simulink model "EST"  (R2025a)
settings: Solver=FixedStepAuto  StartTime=0.0  StopTime=31536000  FixedStep=deltat  MaxStep=0.05  RelTol=1e-3
values from neighbouring files (symbols this model uses):
  A_tank = 6*pi*r_tank^2    [preprocessing.m]
  C_s = m_ads*c_ads + m_w_min*c_w + m_tank*c_tank    [preprocessing.m]
  deltaH = 2.579E6*unit("J")/unit("kg")    [preprocessing.m]
  efficiencyBattery = 0.90    (= 0.9)    [preprocessing.m]
  efficiencyHeater = 1.00    (= 1)    [preprocessing.m]
  EStorageInitial = 2.0*unit("kWh")    [preprocessing.m]
  k_0 = (15*D_0)/(d_p/2)^2    [preprocessing.m]
  m_eq = m_w_max    [preprocessing.m]
  m_w_0 = m_w_min    [preprocessing.m]
  m_w_min = X_min*m_ads    [preprocessing.m]
  Max_Capacity_J = volumes_m3(k) * energy_density * conversion_factor    [optimalization.m]    (also in preprocessing.m = EStorageMax)
  R = 8.314*unit("J")/(unit("mol")*unit("K"))    [preprocessing.m]
  R_cable = L_cable*Rprime_cable    [preprocessing.m]
  T_ambient = (8+273.15)*unit("K")    [preprocessing.m]
  T_s_0 = T_ambient    [preprocessing.m]
  T_w = (50+273.15)*unit("K")    [preprocessing.m]
  U_tank = 1 / (1/h_inside + t_wall/k_steel + 1/h_outside)    [preprocessing.m]
  UA_pipe = U_pipe*A_pipe    [preprocessing.m]
  V_system = 400    [preprocessing.m]
settings Model: Creator=joche  LastModifiedBy=20253351
settings DataIOCC: SaveFormat=Array  SaveOutput=off  ReturnWorkspaceOutputs=off
settings OptimizationCC: ReuseModelBlockBuffer=off
settings ModelReferenceCC: EnableRefExpFcnMdlSchedulingChecks=on
settings RTWCC: GPUComputeCapability=3.5

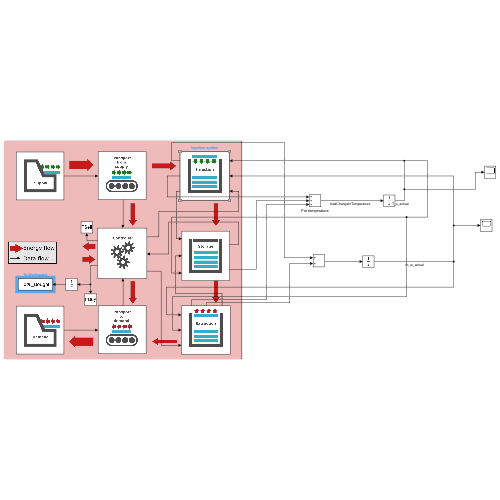
[thumbnail: Simulink's stored preview of the top-level diagram]
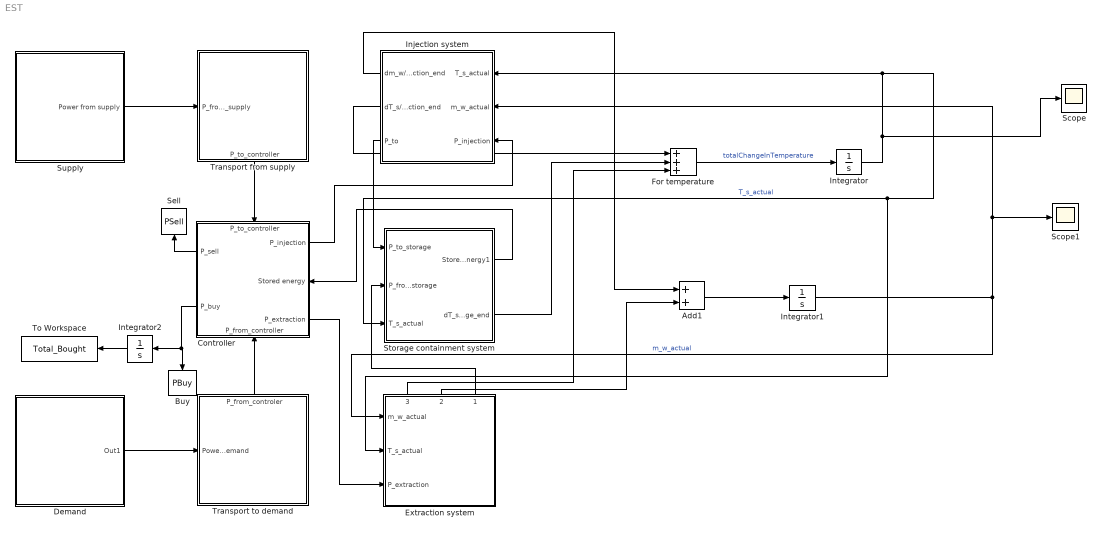
== system EST ==
  Add1 : Sum
  Buy : ToWorkspace  VariableName=PBuy  SampleTime=-1
  Controller : Subsystem
      settings: PortSchema="{\"entries\":[{\"content\":{\"sides\":[{\"content\":{\"connectorIds\":[\"Out3\",\"Out4\"]},\"type\":\"ConnectorPlacement.EquallySpacedRectSide\",\"uuid\":\"4daf33ce-c96a-4783-b5c4-228eed953e01\"},{\"content\":{\"connectorIds\":[\"Out1\",\"In3\",\"Out2\"],\"side\":\"RIGHT\"},\"type\":\"ConnectorPlacement.EquallySpacedRectSide\",\"uuid\":\"e9942e50-8467-4af8-b79b-80636cbc76e5\"},{\"content\":{\"connectorIds\":[\"In1\"],\"side\":\"TOP\"},\"type\":\"ConnectorPlacement.EquallySpacedRectSide\",\"uuid\":\"f315e931-d69b-4751-b712-f89c6c81baeb\"},{\"content\":{\"connectorIds\":[\"In2\"],\"side\":\"BOTTOM\"},\"type\":\"ConnectorPlacement.EquallySpacedRectSide\",\"uuid\":\"44715ee6-5cd5-4669-bcb9-5ed7c869bdb3\"}]},\"type\":\"ConnectorPlacement.EquallySpacedConnector\",\"uuid\":\"fff48899-944b-4064-b7d7-ecc12144fb48\"}],\"packageUris\":[\"http://schema.mathworks.com/mf0/Connector/R2020b\"],\"version\":\"1.0\"}"
      mask Display: image('$imagefile'); % Use "Edit Image" on toolstrip to change.
  Demand : Subsystem
      mask Display: image('$imagefile'); % Use "Edit Image" on toolstrip to change.
  Extraction system : Subsystem
      settings: PortSchema="{\"entries\":[{\"content\":{\"sides\":[{\"content\":{},\"type\":\"ConnectorPlacement.EquallySpacedRectSide\",\"uuid\":\"05c5933d-55fc-4e06-853f-fc26d42905f9\"},{\"content\":{\"connectorIds\":[\"In1\",\"In2\",\"In3\"],\"side\":\"RIGHT\"},\"type\":\"ConnectorPlacement.EquallySpacedRectSide\",\"uuid\":\"327426c5-31d5-498b-a2bd-83e49353408c\"},{\"content\":{\"side\":\"TOP\"},\"type\":\"ConnectorPlacement.EquallySpacedRectSide\",\"uuid\":\"55306cf3-a3de-4385-a5ae-b8600ecdd5a2\"},{\"content\":{\"connectorIds\":[\"Out1\",\"Out2\",\"Out3\"],\"side\":\"BOTTOM\"},\"type\":\"ConnectorPlacement.EquallySpacedRectSide\",\"uuid\":\"08fcc9c3-40d3-4ac6-b914-dfeef6039ffb\"}]},\"type\":\"ConnectorPlacement.EquallySpacedConnector\",\"uuid\":\"cb35d5ba-e8c6-462c-b7b2-fe8356d4b0a1\"}],\"packageUris\":[\"http://schema.mathworks.com/mf0/Connector/R2020b\"],\"version\":\"1.0\"}"
      mask Display: image('$imagefile'); % Use "Edit Image" on toolstrip to change.
  For temperature : Sum  Inputs=+++
  Injection system : Subsystem
      mask Display: image('$imagefile'); % Use "Edit Image" on toolstrip to change.
  Integrator : Integrator  InitialCondition=T_s_0
  Integrator1 : Integrator  InitialCondition=m_w_0
  Integrator2 : Integrator
  Scope : Scope
      settings: ActiveDisplayYMinimum=-1  ActiveDisplayYMaximum=1  DataLoggingVariableName=ScopeData7
  Scope1 : Scope
      settings: ActiveDisplayYMinimum=-895.99568542877842  ActiveDisplayYMaximum=10043.823661162089  DataLoggingVariableName=ScopeData8
  Sell : ToWorkspace  VariableName=PSell  SampleTime=-1
  Storage containment system : Subsystem
      mask Display: image('$imagefile'); % Use "Edit Image" on toolstrip to change.
  Supply : Subsystem
      mask Display: image('$imagefile'); % Use "Edit Image" on toolstrip to change.
  To Workspace : ToWorkspace  VariableName=Total_Bought  SaveFormat=Timeseries  SampleTime=-1
  Transport from supply : Subsystem
      settings: PortSchema="{\"entries\":[{\"content\":{\"sides\":[{\"content\":{\"connectorIds\":[\"In1\"]},\"type\":\"ConnectorPlacement.EquallySpacedRectSide\",\"uuid\":\"31329006-3d36-4d93-9c44-7503a515d397\"},{\"content\":{\"connectorIds\":[],\"side\":\"RIGHT\"},\"type\":\"ConnectorPlacement.EquallySpacedRectSide\",\"uuid\":\"aba139c7-f9b6-4881-a56b-a4cbbedacd88\"},{\"content\":{\"connectorIds\":[],\"side\":\"TOP\"},\"type\":\"ConnectorPlacement.EquallySpacedRectSide\",\"uuid\":\"e683eb73-7a35-4160-9c39-da83856a6278\"},{\"content\":{\"connectorIds\":[\"Out1\"],\"side\":\"BOTTOM\"},\"type\":\"ConnectorPlacement.EquallySpacedRectSide\",\"uuid\":\"1170dd18-447c-437f-9043-6812c2877331\"}]},\"type\":\"ConnectorPlacement.EquallySpacedConnector\",\"uuid\":\"804af608-1d70-444f-af69-e05f19bf98f3\"}],\"packageUris\":[\"http://schema.mathworks.com/mf0/Connector/R2020b\"],\"version\":\"1.0\"}"
      mask Display: image('$imagefile'); % Use "Edit Image" on toolstrip to change.
  Transport to demand : Subsystem
      settings: PortSchema="{\"entries\":[{\"content\":{\"sides\":[{\"content\":{\"connectorIds\":[\"In1\"]},\"type\":\"ConnectorPlacement.EquallySpacedRectSide\",\"uuid\":\"31329006-3d36-4d93-9c44-7503a515d397\"},{\"content\":{\"connectorIds\":[],\"side\":\"RIGHT\"},\"type\":\"ConnectorPlacement.EquallySpacedRectSide\",\"uuid\":\"aba139c7-f9b6-4881-a56b-a4cbbedacd88\"},{\"content\":{\"connectorIds\":[\"Out1\"],\"side\":\"TOP\"},\"type\":\"ConnectorPlacement.EquallySpacedRectSide\",\"uuid\":\"e683eb73-7a35-4160-9c39-da83856a6278\"},{\"content\":{\"connectorIds\":[],\"side\":\"BOTTOM\"},\"type\":\"ConnectorPlacement.EquallySpacedRectSide\",\"uuid\":\"c378138f-7233-4483-870c-40a69b3495ee\"}]},\"type\":\"ConnectorPlacement.EquallySpacedConnector\",\"uuid\":\"804af608-1d70-444f-af69-e05f19bf98f3\"}],\"packageUris\":[\"http://schema.mathworks.com/mf0/Connector/R2020b\"],\"version\":\"1.0\"}"
      mask Display: image('$imagefile'); % Use "Edit Image" on toolstrip to change.
  wires:
  Supply/1(Power from supply) -> Transport from supply/1(P_from_supply)
  Transport from supply/1(P_to_controller) -> Controller/1(P_to_controller)
  Transport to demand/1(P_from_controler) -> Controller/2(P_from_controller)
  Demand/1(Out1) -> Transport to demand/1(Power to demand)
  Controller/3(P_sell) -> Sell/1
  Controller/2(P_extraction) -> Extraction system/1(P_extraction)
  Injection system/1(P_to) -> Storage containment system/1(P_to_storage)
  Extraction system/1(P_from_storage) -> Storage containment system/2(P_from_storage)
  Storage containment system/1(Stored energy1) -> Controller/3(Stored energy)
  Controller/1(P_injection) -> Injection system/1(P_injection)
  Controller/4(P_buy) -> Integrator2/1, Buy/1
  Injection system/2(dT_s/dt_injection_end) -> For temperature/1
  Storage containment system/2(dT_s/dt_storage_end) -> For temperature/2
  Extraction system/3(dT_s/dt_end_extraction) -> For temperature/3
  For temperature/1 -> Integrator/1  "totalChangeInTemperature"
  Integrator/1 -> Scope/1, Injection system/3(T_s_actual), Extraction system/2(T_s_actual), Storage containment system/3(T_s_actual)  "T_s_actual"
  Injection system/3(dm_w/dt_injection_end) -> Add1/1
  Extraction system/2(dm_w/dt_end_extraction) -> Add1/2
  Add1/1 -> Integrator1/1
  Integrator1/1 -> Scope1/1, Injection system/2(m_w_actual), Extraction system/3(m_w_actual)  "m_w_actual"
  Integrator2/1 -> To Workspace/1

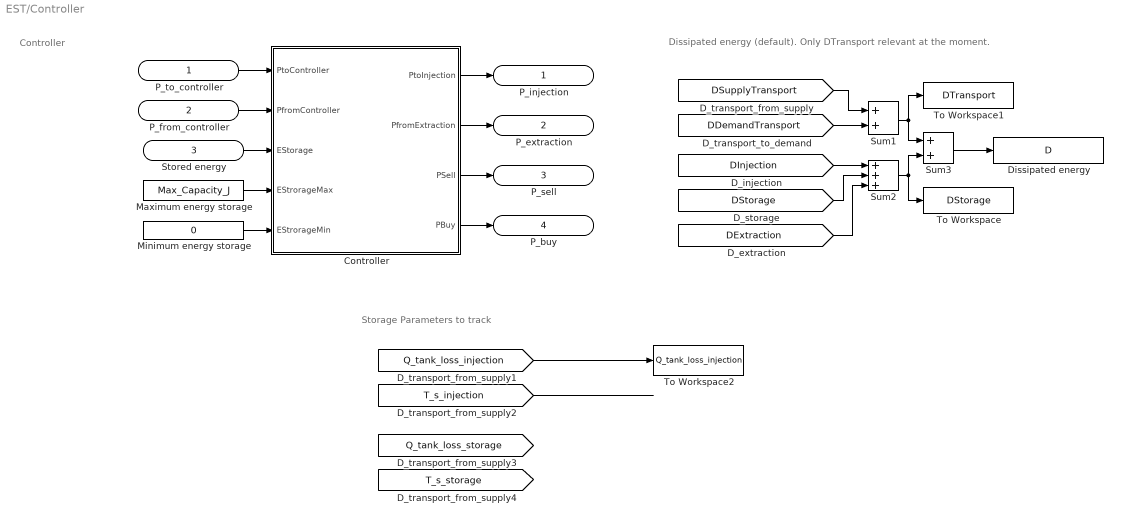
== system EST/Controller ==
  note: Dissipated energy (default). Only DTransport relevant at the moment.
  note: Controller
  note: Storage Parameters to track
  P_to_controller : Inport
  P_from_controller : Inport  Port=2
  Stored energy : Inport  Port=3
  Controller : MATLAB Function  TreatAsAtomicUnit=on
  Dissipated energy : ToWorkspace  VariableName=D  SampleTime=-1
  Maximum energy storage : Constant  Value=Max_Capacity_J
  Minimum energy storage : Constant  Value=0
  Sum1 : Sum
  Sum2 : Sum  Inputs=+++
  Sum3 : Sum
  To Workspace : ToWorkspace  VariableName=DStorage  SampleTime=-1
  To Workspace1 : ToWorkspace  VariableName=DTransport  SampleTime=-1
  To Workspace2 : ToWorkspace  VariableName=Q_tank_loss_injection  SaveFormat=Timeseries  SampleTime=-1
  P_injection : Outport
  P_extraction : Outport  Port=2
  P_sell : Outport  Port=3
  P_buy : Outport  Port=4
  wires:
  P_from_controller/1 -> Controller/2(PfromController)
  Controller/2(PfromExtraction) -> P_extraction/1
  Controller/3(PSell) -> P_sell/1
  Controller/4(PBuy) -> P_buy/1
  Minimum energy storage/1 -> Controller/5(EStrorageMin)
  Maximum energy storage/1 -> Controller/4(EStrorageMax)
  P_to_controller/1 -> Controller/1(PtoController)
  Controller/1(PtoInjection) -> P_injection/1
  Stored energy/1 -> Controller/3(EStorage)
  [DDemandTransport] -> Sum1/2
  [DSupplyTransport] -> Sum1/1
  [DInjection] -> Sum2/1
  [DStorage] -> Sum2/2
  [DExtraction] -> Sum2/3
  Sum2/1 -> To Workspace/1, Sum3/2
  Sum1/1 -> To Workspace1/1, Sum3/1
  Sum3/1 -> Dissipated energy/1
  [Q_tank_loss_injection] -> To Workspace2/1
  [T_s_injection] -> ?

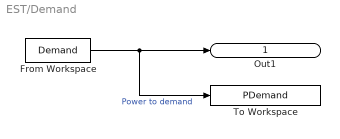
== system EST/Demand ==
  From Workspace : FromWorkspace  VariableName=Demand  OutputAfterFinalValue=Setting to zero
  To Workspace : ToWorkspace  VariableName=PDemand  SampleTime=-1
  Out1 : Outport
  wires:
  From Workspace/1 -> To Workspace/1, Out1/1  "Power to demand"

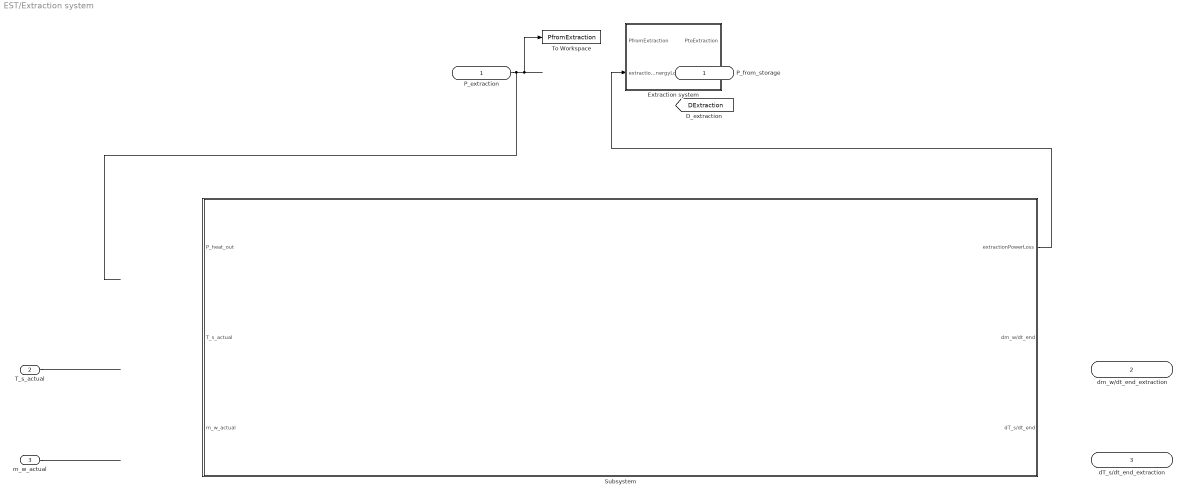
== system EST/Extraction system ==
  P_extraction : Inport
  T_s_actual : Inport  Port=2
  m_w_actual : Inport  Port=3
  Extraction system : MATLAB Function  TreatAsAtomicUnit=on
  Subsystem : Subsystem
  To Workspace : ToWorkspace  VariableName=PfromExtraction  SampleTime=-1
  P_from_storage : Outport
  dm_w/dt_end_extraction : Outport  Port=2
  dT_s/dt_end_extraction : Outport  Port=3
  tag scope: DExtraction=global
  wires:
  P_extraction/1 -> To Workspace/1
  ? -> P_from_storage/1
  ? -> [DExtraction]
  Subsystem/1(extractionPowerLoss) -> Extraction system/2(extractionEnergyLoss)
  ? -> dm_w/dt_end_extraction/1
  ? -> dT_s/dt_end_extraction/1
  T_s_actual/1 -> ?
  m_w_actual/1 -> ?

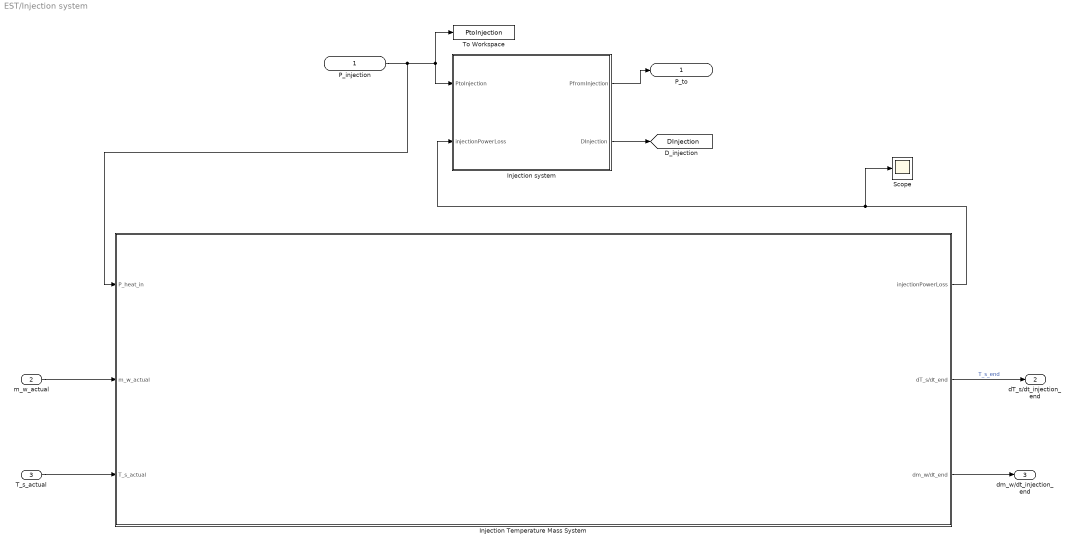
== system EST/Injection system ==
  P_injection : Inport
  m_w_actual : Inport  Port=2
  T_s_actual : Inport  Port=3
  Injection Temperature Mass System : Subsystem
  Injection system : MATLAB Function  TreatAsAtomicUnit=on
  Scope : Scope
      settings: ActiveDisplayYMinimum=-7184.0347360498881  ActiveDisplayYMaximum=5973.1294987784431  DataLoggingVariableName=ScopeData9
  To Workspace : ToWorkspace  VariableName=PtoInjection  SampleTime=-1
  P_to : Outport
  dT_s/dt_injection_end : Outport  Port=2
  dm_w/dt_injection_end : Outport  Port=3
  tag scope: DInjection=global
  wires:
  P_injection/1 -> Injection Temperature Mass System/1(P_heat_in), Injection system/1(PtoInjection), To Workspace/1
  Injection system/2(DInjection) -> [DInjection]
  Injection system/1(PfromInjection) -> P_to/1
  Injection Temperature Mass System/1(injectionPowerLoss) -> Scope/1, Injection system/2(injectionPowerLoss)
  Injection Temperature Mass System/3(dm_w/dt_end) -> dm_w/dt_injection_end/1
  Injection Temperature Mass System/2(dT_s/dt_end) -> dT_s/dt_injection_end/1  "T_s_end"
  m_w_actual/1 -> Injection Temperature Mass System/2(m_w_actual)
  T_s_actual/1 -> Injection Temperature Mass System/3(T_s_actual)

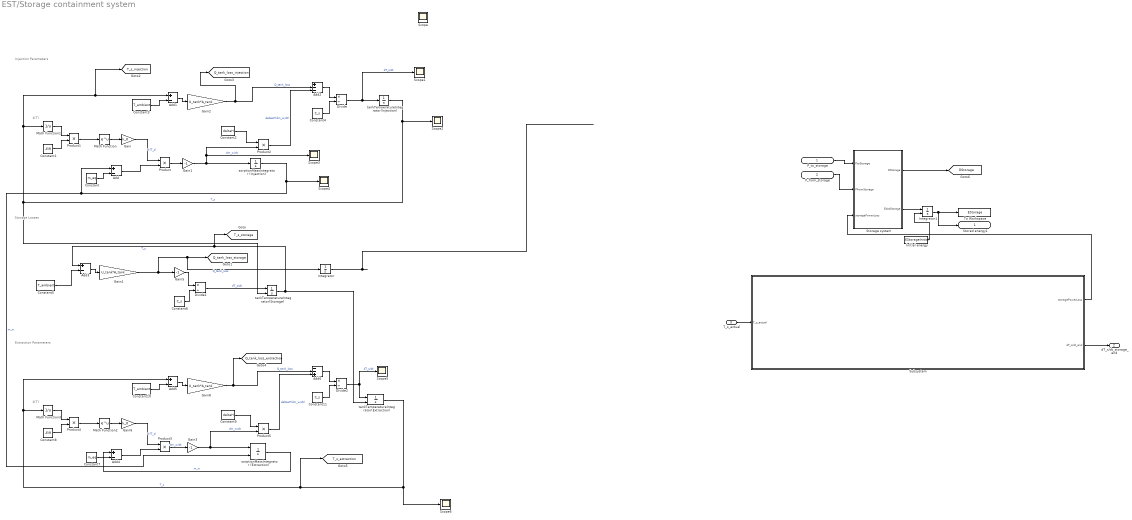
== system EST/Storage containment system ==
  note: Storage Losses
  note: Injection Parameters
  note: k(T)
  note: k(T)
  note: Extraction Parameters
  P_to_storage : Inport
  P_from_storage : Inport  Port=2
  T_s_actual : Inport  Port=3
  Add{,1,3..5} (5 alike) : Sum  Inputs=+-
  Add2 : Sum  Inputs=+--
  Add6 : Sum  Inputs=--+
  Constant : Constant  Value=m_eq
  Constant1 : Constant  Value=-E/R
  Constant10 : Constant  Value=T_ambient
  Constant11 : Constant  Value=C_s
  Constant2 : Constant  Value=deltaH
  Constant3 : Constant  Value=T_ambient
  Constant4 : Constant  Value=C_s
  Constant5 : Constant  Value=T_ambient
  Constant6 : Constant  Value=C_s
  Constant7 : Constant  Value=m_eq
  Constant8 : Constant  Value=-E/R
  Constant9 : Constant  Value=deltaH
  Divide : Product  Inputs=*/
  Divide1 : Product  Inputs=*/
  Divide2 : Product  Inputs=*/
  Gain : Gain  Gain=k_0
  Gain1 : Gain  Gain=-1
  Gain2 : Gain  Gain=U_tank*A_tank
  Gain3 : Gain  Gain=-1
  Gain4 : Gain  Gain=U_tank*A_tank
  Gain5 : Gain  Gain=-1
  Gain6 : Gain  Gain=k_0
  Gain8 : Gain  Gain=U_tank*A_tank
  Initial energy : Constant  Value=EStorageInitial
  Integrator : Integrator
  Integrator1 : Integrator  InitialConditionSource=external
  Math Function : Math
  Math Function1 : Math  Operator=reciprocal
  Math Function2 : Math
  Math Function3 : Math  Operator=reciprocal
  Product{,1..5} (6 alike) : Product
  Scope{,1..6} (7 alike) : Scope
      Scope settings: ActiveDisplayYMinimum=-1  ActiveDisplayYMaximum=1
      Scope1 settings: ActiveDisplayYMinimum=-4.0765015018520045E-5  ActiveDisplayYMaximum=2.1866995862680802E-5
      Scope2 settings: ActiveDisplayYMinimum=281.007353821474  ActiveDisplayYMaximum=289.04893636017056  DataLoggingVariableName=ScopeData2
      Scope3 settings: ActiveDisplayYMinimum=-0.027590583189522518  ActiveDisplayYMaximum=0.24831524870571758  DataLoggingVariableName=ScopeData3
      Scope4 settings: ActiveDisplayYMinimum=-486.81818181817505  ActiveDisplayYMaximum=8963.18181818176  DataLoggingVariableName=ScopeData4
      Scope5 settings: ActiveDisplayYMinimum=-1  ActiveDisplayYMaximum=1  DataLoggingVariableName=ScopeData5
      Scope6 settings: ActiveDisplayYMinimum=-4.2911297495566172E+12  ActiveDisplayYMaximum=4.7679219482562183E+11  DataLoggingVariableName=ScopeData6
  Storage system : MATLAB Function  TreatAsAtomicUnit=on
  Subsystem : Subsystem
  To Workspace : ToWorkspace  VariableName=EStorage  SampleTime=-1
  sorptionMassIntegrator (Extraction) : Integrator  InitialConditionSource=external  InitialCondition=m_w_0  LimitOutput=on  LowerSaturationLimit=m_w_min
  sorptionMassIntegrator (Injection) : Integrator  InitialCondition=m_w_0  LimitOutput=on  LowerSaturationLimit=m_w_min
  tankTemperatureIntegrator(Extraction) : Integrator  InitialConditionSource=external  InitialCondition=T_s_0  LimitOutput=on
  tankTemperatureIntegrator(Injection) : Integrator  InitialCondition=T_s_0  LimitOutput=on
  tankTemperatureIntegrator(Storage) : Integrator  InitialConditionSource=external  InitialCondition=T_s_0
  Stored energy1 : Outport
  dT_s/dt_storage_end : Outport  Port=2
  tag scope: DStorage=global, Q_tank_loss_extraction=global, Q_tank_loss_injection=global, Q_tank_loss_storage=global, T_s_extraction=global, T_s_injection=global, T_s_storage=global
  wires:
  P_to_storage/1 -> Storage system/1(PtoStorage)
  P_from_storage/1 -> Storage system/2(PfromStorage)
  Add3/1 -> Gain4/1
  Constant5/1 -> Add3/2
  Constant6/1 -> Divide1/2
  Gain5/1 -> Divide1/1
  Divide1/1 -> tankTemperatureIntegrator(Storage)/1  "dT_s/dt"
  Gain4/1 -> [Q_tank_loss_storage], Integrator/1, Gain5/1  "Q_tank_loss"
  tankTemperatureIntegrator(Storage)/1 -> [T_s_storage], Add3/1, tankTemperatureIntegrator(Extraction)/2  "T_s"
  Storage system/2(EdotStorage) -> Integrator1/1
  Initial energy/1 -> Integrator1/2
  Integrator1/1 -> Stored energy1/1, To Workspace/1
  Integrator/1 -> ?
  tankTemperatureIntegrator(Injection)/1 -> tankTemperatureIntegrator(Storage)/2, [T_s_injection], Add1/1, Math Function1/1, Scope2/1  "T_s"
  Constant10/1 -> Add5/2
  Add5/1 -> Gain8/1
  tankTemperatureIntegrator(Extraction)/1 -> [T_s_extraction], Add5/1, Math Function3/1, Scope6/1  "T_s"
  Product3/1 -> Gain3/1  "dm_w/dt"
  Divide2/1 -> Scope5/1, tankTemperatureIntegrator(Extraction)/1  "dT_s/dt"
  Add4/1 -> Product3/2
  Math Function3/1 -> Product4/1
  Constant11/1 -> Divide2/2
  Constant7/1 -> Add4/2
  Constant9/1 -> Product5/1
  Gain6/1 -> Product3/1  "k(T_s)"
  Add6/1 -> Divide2/1
  Product5/1 -> Add6/3  "deltaH*(dm_w/dt)"
  Constant8/1 -> Product4/2
  Math Function2/1 -> Gain6/1
  Product4/1 -> Math Function2/1
  Gain8/1 -> Add6/2, [Q_tank_loss_extraction]  "Q_tank_loss"
  sorptionMassIntegrator (Extraction)/1 -> Add4/1  "m_w"
  Gain3/1 -> Product5/2, sorptionMassIntegrator (Extraction)/1  "dm_w/dt"
  Constant3/1 -> Add1/2
  Add1/1 -> Gain2/1
  Gain2/1 -> [Q_tank_loss_injection], Add2/2  "Q_tank_loss"
  Product2/1 -> Add2/3  "deltaH*(dm_w/dt)"
  Constant2/1 -> Product2/1
  Gain1/1 -> Scope3/1, Product2/2, sorptionMassIntegrator (Injection)/1  "dm_w/dt"
  sorptionMassIntegrator (Injection)/1 -> Scope4/1, sorptionMassIntegrator (Extraction)/2, Add/1  "m_w"
  Constant/1 -> Add/2
  Add/1 -> Product/2
  Product/1 -> Gain1/1
  Gain/1 -> Product/1  "k(T_s)"
  Math Function/1 -> Gain/1
  Product1/1 -> Math Function/1
  Math Function1/1 -> Product1/1
  Constant1/1 -> Product1/2
  Add2/1 -> Divide/1
  Constant4/1 -> Divide/2
  Divide/1 -> Scope1/1, tankTemperatureIntegrator(Injection)/1  "dT_s/dt"
  Storage system/1(DStorage) -> [DStorage]
  Subsystem/2(dT_s/dt_end) -> dT_s/dt_storage_end/1
  Subsystem/1(storagePowerLoss) -> Storage system/3(storagePowerLoss)
  T_s_actual/1 -> Subsystem/1(T_s_actual)

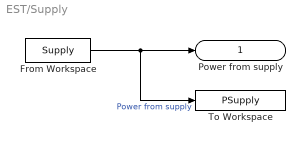
== system EST/Supply ==
  From Workspace : FromWorkspace  VariableName=Supply  OutputAfterFinalValue=Setting to zero
  To Workspace : ToWorkspace  VariableName=PSupply  SampleTime=-1
  Power from supply : Outport
  wires:
  From Workspace/1 -> To Workspace/1, Power from supply/1  "Power from supply"

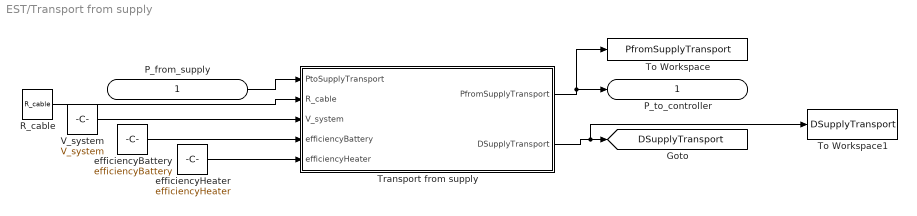
== system EST/Transport from supply ==
  P_from_supply : Inport
  R_cable : Constant  Value=R_cable
  To Workspace : ToWorkspace  VariableName=PfromSupplyTransport  SampleTime=-1
  To Workspace1 : ToWorkspace  VariableName=DSupplyTransport  SampleTime=-1
  Transport from supply : MATLAB Function  TreatAsAtomicUnit=on
  V_system : Constant  Value=V_system
  efficiencyBattery : Constant  Value=efficiencyBattery
  efficiencyHeater : Constant  Value=efficiencyHeater
  P_to_controller : Outport
  tag scope: DSupplyTransport=global
  wires:
  R_cable/1 -> Transport from supply/2(R_cable)
  P_from_supply/1 -> Transport from supply/1(PtoSupplyTransport)
  Transport from supply/1(PfromSupplyTransport) -> To Workspace/1, P_to_controller/1
  Transport from supply/2(DSupplyTransport) -> To Workspace1/1, [DSupplyTransport]
  V_system/1 -> Transport from supply/3(V_system)
  efficiencyBattery/1 -> Transport from supply/4(efficiencyBattery)
  efficiencyHeater/1 -> Transport from supply/5(efficiencyHeater)

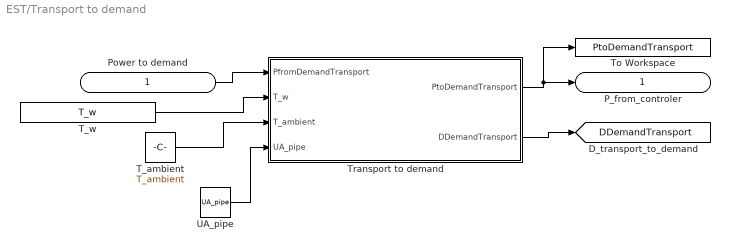
== system EST/Transport to demand ==
  Power to demand : Inport
  T_ambient : Constant  Value=T_ambient
  T_w : Constant  Value=T_w
  To Workspace : ToWorkspace  VariableName=PtoDemandTransport  SampleTime=-1
  Transport to demand : MATLAB Function  TreatAsAtomicUnit=on
  UA_pipe : Constant  Value=UA_pipe
  P_from_controler : Outport
  tag scope: DDemandTransport=global
  wires:
  T_w/1 -> Transport to demand/2(T_w)
  Power to demand/1 -> Transport to demand/1(PfromDemandTransport)
  Transport to demand/1(PtoDemandTransport) -> To Workspace/1, P_from_controler/1
  Transport to demand/2(DDemandTransport) -> [DDemandTransport]
  T_ambient/1 -> Transport to demand/3(T_ambient)
  UA_pipe/1 -> Transport to demand/4(UA_pipe)

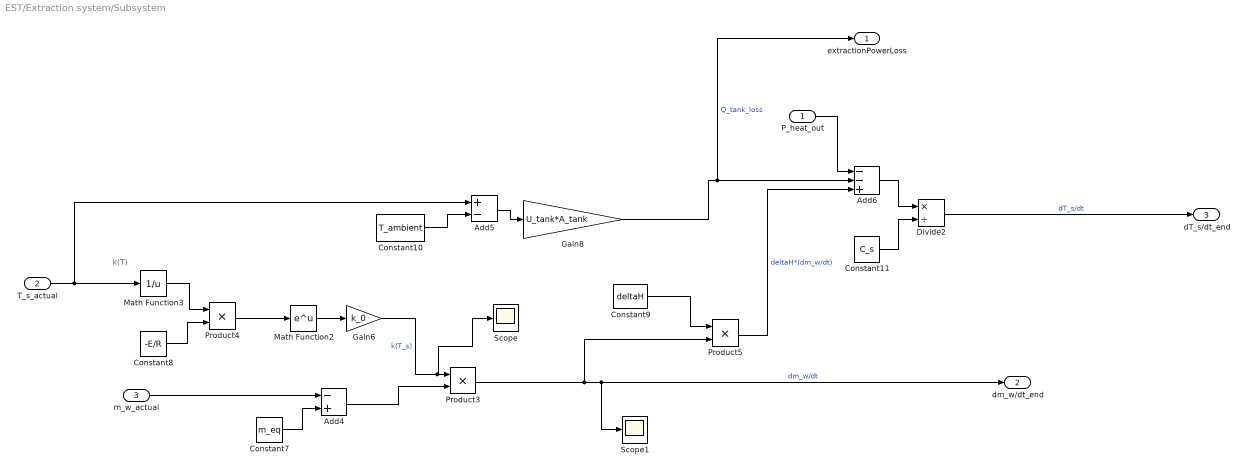
== system EST/Extraction system/Subsystem ==
  note: k(T)
  P_heat_out : Inport
  T_s_actual : Inport  Port=2
  m_w_actual : Inport  Port=3
  Add4 : Sum  Inputs=-+
  Add5 : Sum  Inputs=+-
  Add6 : Sum  Inputs=--+
  Constant10 : Constant  Value=T_ambient
  Constant11 : Constant  Value=C_s
  Constant7 : Constant  Value=m_eq
  Constant8 : Constant  Value=-E/R
  Constant9 : Constant  Value=deltaH
  Divide2 : Product  Inputs=*/
  Gain6 : Gain  Gain=k_0
  Gain8 : Gain  Gain=U_tank*A_tank
  Math Function2 : Math
  Math Function3 : Math  Operator=reciprocal
  Product3 : Product
  Product4 : Product
  Product5 : Product
  Scope : Scope
      settings: ActiveDisplayYMinimum=-1  ActiveDisplayYMaximum=1  DataLoggingVariableName=ScopeData10
  Scope1 : Scope
      settings: ActiveDisplayYMinimum=-1  ActiveDisplayYMaximum=1  DataLoggingVariableName=ScopeData11
  extractionPowerLoss : Outport
  dm_w/dt_end : Outport  Port=2
  dT_s/dt_end : Outport  Port=3
  wires:
  Add4/1 -> Product3/2
  Divide2/1 -> dT_s/dt_end/1  "dT_s/dt"
  Constant9/1 -> Product5/1
  Math Function2/1 -> Gain6/1
  Add5/1 -> Gain8/1
  Constant7/1 -> Add4/2
  Gain8/1 -> extractionPowerLoss/1, Add6/2  "Q_tank_loss"
  Constant10/1 -> Add5/2
  Add6/1 -> Divide2/1
  Product3/1 -> dm_w/dt_end/1, Scope1/1, Product5/2  "dm_w/dt"
  Product5/1 -> Add6/3  "deltaH*(dm_w/dt)"
  Product4/1 -> Math Function2/1
  Gain6/1 -> Scope/1, Product3/1  "k(T_s)"
  Constant8/1 -> Product4/2
  Constant11/1 -> Divide2/2
  Math Function3/1 -> Product4/1
  P_heat_out/1 -> Add6/1
  T_s_actual/1 -> Math Function3/1, Add5/1
  m_w_actual/1 -> Add4/1

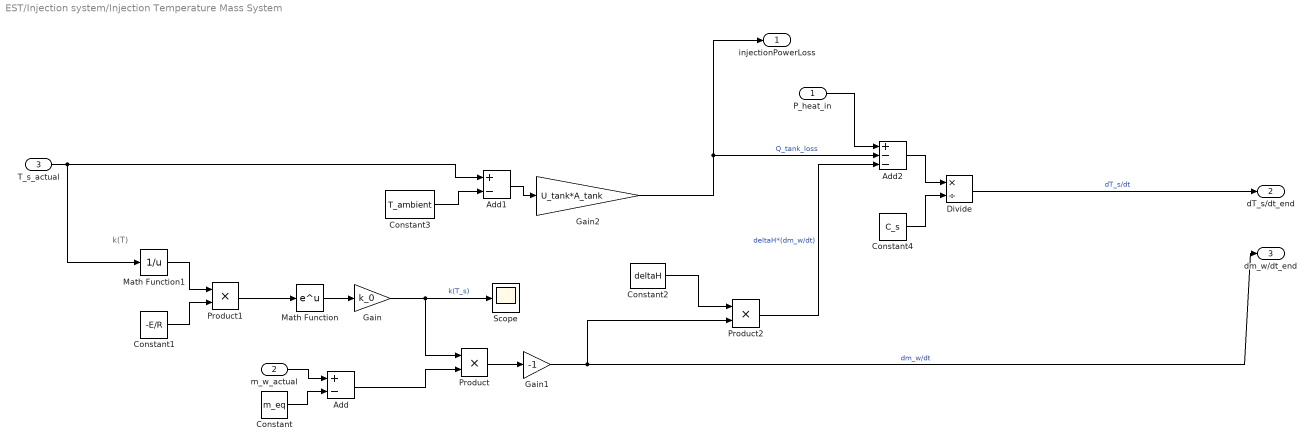
== system EST/Injection system/Injection Temperature Mass System ==
  note: k(T)
  P_heat_in : Inport
  m_w_actual : Inport  Port=2
  T_s_actual : Inport  Port=3
  Add : Sum  Inputs=+-
  Add1 : Sum  Inputs=+-
  Add2 : Sum  Inputs=+--
  Constant : Constant  Value=m_eq
  Constant1 : Constant  Value=-E/R
  Constant2 : Constant  Value=deltaH
  Constant3 : Constant  Value=T_ambient
  Constant4 : Constant  Value=C_s
  Divide : Product  Inputs=*/
  Gain : Gain  Gain=k_0
  Gain1 : Gain  Gain=-1
  Gain2 : Gain  Gain=U_tank*A_tank
  Math Function : Math
  Math Function1 : Math  Operator=reciprocal
  Product : Product
  Product1 : Product
  Product2 : Product
  Scope : Scope
      settings: ActiveDisplayYMinimum=2.9002792603777036E-5  ActiveDisplayYMaximum=2.9357228982545738E-5  DataLoggingVariableName=ScopeData12
  injectionPowerLoss : Outport
  dT_s/dt_end : Outport  Port=2
  dm_w/dt_end : Outport  Port=3
  wires:
  Constant/1 -> Add/2
  Product/1 -> Gain1/1
  Constant4/1 -> Divide/2
  Divide/1 -> dT_s/dt_end/1  "dT_s/dt"
  Add/1 -> Product/2
  Gain1/1 -> dm_w/dt_end/1, Product2/2  "dm_w/dt"
  Gain2/1 -> injectionPowerLoss/1, Add2/2  "Q_tank_loss"
  Add1/1 -> Gain2/1
  Constant2/1 -> Product2/1
  Constant3/1 -> Add1/2
  Add2/1 -> Divide/1
  Constant1/1 -> Product1/2
  Product1/1 -> Math Function/1
  Math Function1/1 -> Product1/1
  Gain/1 -> Product/1, Scope/1  "k(T_s)"
  Math Function/1 -> Gain/1
  Product2/1 -> Add2/3  "deltaH*(dm_w/dt)"
  P_heat_in/1 -> Add2/1
  m_w_actual/1 -> Add/1
  T_s_actual/1 -> Math Function1/1, Add1/1

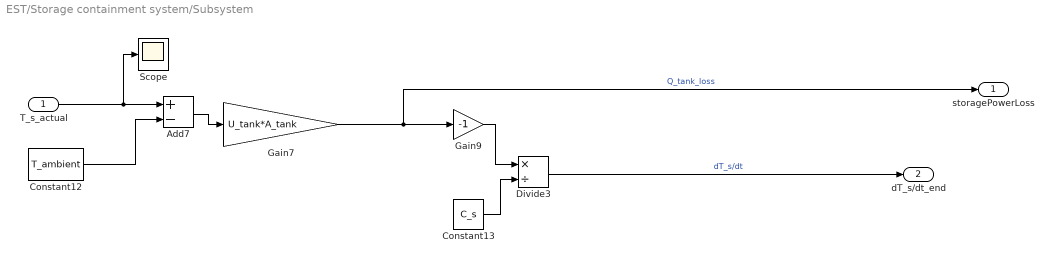
== system EST/Storage containment system/Subsystem ==
  T_s_actual : Inport
  Add7 : Sum  Inputs=+-
  Constant12 : Constant  Value=T_ambient
  Constant13 : Constant  Value=C_s
  Divide3 : Product  Inputs=*/
  Gain7 : Gain  Gain=U_tank*A_tank
  Gain9 : Gain  Gain=-1
  Scope : Scope
      settings: ActiveDisplayYMinimum=271.84963832409619  ActiveDisplayYMaximum=289.64119142300439  DataLoggingVariableName=ScopeData13
  storagePowerLoss : Outport
  dT_s/dt_end : Outport  Port=2
  wires:
  Divide3/1 -> dT_s/dt_end/1  "dT_s/dt"
  Constant13/1 -> Divide3/2
  Gain9/1 -> Divide3/1
  Gain7/1 -> storagePowerLoss/1, Gain9/1  "Q_tank_loss"
  Add7/1 -> Gain7/1
  Constant12/1 -> Add7/2
  T_s_actual/1 -> Scope/1, Add7/1

== matlab function EST/Injection system/Injection system ==
  data: PtoInjection input; PfromInjection output; DInjection output; injectionPowerLoss input
function [PfromInjection, DInjection] = injection(PtoInjection, injectionPowerLoss)
    DInjection = injectionPowerLoss;
    PfromInjection = PtoInjection - DInjection;

== matlab function EST/Transport from supply/Transport from supply ==
  data: PtoSupplyTransport input; PfromSupplyTransport output; R_cable input; DSupplyTransport output; V_system input; efficiencyBattery input; efficiencyHeater input
function [PfromSupplyTransport, DSupplyTransport] = supplyTransport( ...
    PtoSupplyTransport, R_cable, V_system, efficiencyBattery, efficiencyHeater)

% Physical transport model from supply to injection/storage.
% Cable losses are calculated using Joule heating:
% P_loss = R_cable * I^2, where I = P/V.
% Battery and heater are represented by efficiency factors.

    Pin = max(PtoSupplyTransport, 0);

    I_cable = Pin / V_system;

    P_loss_cable = R_cable * I_cable^2;

    P_after_cable = max(Pin - P_loss_cable, 0);

    P_after_battery = efficiencyBattery * P_after_cable;

    PfromSupplyTransport = efficiencyHeater * P_after_battery;

    DSupplyTransport = Pin - PfromSupplyTransport;

end

== matlab function EST/Controller/Controller ==
  data: PtoInjection output; PfromExtraction output; PSell output; PBuy output; PtoController input; PfromController input; EStorage input; EStrorageMax input; EStrorageMin input
function [PtoInjection, PfromExtraction, PSell, PBuy] = controller(PtoController, PfromController, EStorage, EStrorageMax, EStrorageMin)
    
    %% Power surplus or deficit

    deltaP = PtoController - PfromController;

    % Power surplus
    if deltaP >= 0

        %% Storage injection

        % Storage system is not full
        if EStorage < EStrorageMax 

            PtoInjection = deltaP;

        % Storage system is full
        else
            PtoInjection = 0;
        end

        %% Storage extraction

        PfromExtraction = 0;

        %% Load-balancing
        PSell   = deltaP - PtoInjection;
        PBuy    = 0;

    % Power deficit
    else

        %% Storage injection

        PtoInjection = 0;

        %% Storage extraction

        % Storage system is not empty
        if EStorage > EStrorageMin

            PfromExtraction = -deltaP;

        % Storage system is empty
        else
            PfromExtraction = 0;
        end

        %% Load-balancing

        PSell = 0;
        PBuy  = -deltaP - PfromExtraction;
    end

== matlab function EST/Extraction system/Extraction system ==
  data: PfromExtraction input; PtoExtraction output; extractionEnergyLoss input; DExtraction output
function [PtoExtraction, DExtraction] = extraction(PfromExtraction, extractionEnergyLoss)
    DExtraction = extractionEnergyLoss;
    PtoExtraction = PfromExtraction - DExtraction;

== matlab function EST/Storage containment system/Storage system ==
  data: DStorage output; EdotStorage output; PtoStorage input; PfromStorage input; storagePowerLoss input
function [DStorage, EdotStorage]= Storage(PtoStorage, PfromStorage, storagePowerLoss)
    DStorage = storagePowerLoss;
    EdotStorage = PtoStorage - PfromStorage - storagePowerLoss;

== matlab function EST/Transport to demand/Transport to demand ==
  data: PfromDemandTransport input; PtoDemandTransport output; T_w input; DDemandTransport output; T_ambient input; UA_pipe input
function [PtoDemandTransport, DDemandTransport] = demandTransport( ...
    PfromDemandTransport, T_w, T_ambient, UA_pipe)

% Transport to demand model that is parameter-dependent
% Heat is lost from the hot water pipe to the basement:
% Q_pipe_loss = UA_pipe * (T_w - T_ambient)

    % Available heat from extraction/storage
    P_available = max(PfromDemandTransport, 0);

    % Pipe heat loss to basement
    Q_pipe_loss = UA_pipe * (T_w - T_ambient);

    % Prevent negative loss if temperature assumptions change
    Q_pipe_loss = max(Q_pipe_loss, 0);

    % Useful heat delivered to demand
    PtoDemandTransport = max(P_available - Q_pipe_loss, 0);

    % Total unavailable/lost heat
    DDemandTransport = P_available - PtoDemandTransport;

end
